simulink model "exercicio3lcsd3"  (R2026a)
settings: Solver=VariableStepAuto  MaxStep=1e-3
settings Model: Creator=shumy  LastModifiedBy=shumy

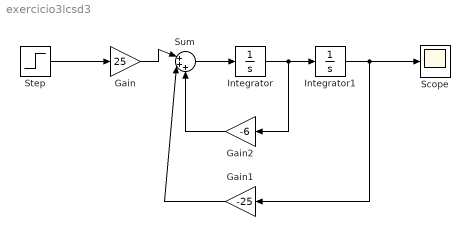
== system exercicio3lcsd3 ==
  Gain : Gain  Gain=25
  Gain1 : Gain  Gain=-25
  Gain2 : Gain  Gain=-6
  Integrator : Integrator
  Integrator1 : Integrator
  Scope : Scope
      settings: ActiveDisplayYMinimum=-0.1368475046086062  ActiveDisplayYMaximum=1.231627541477456
  Step : Step  SampleTime=0
  Sum : Sum  Inputs=|+++
  wires:
  Step/1 -> Gain/1
  Gain/1 -> Sum/1
  Sum/1 -> Integrator/1
  Integrator/1 -> Gain2/1, Integrator1/1
  Integrator1/1 -> Scope/1, Gain1/1
  Gain2/1 -> Sum/3
  Gain1/1 -> Sum/2
